simulink model "rgb_conterller_demo"  (Simulink 7.3)
settings: Solver=ode3  SolverMode=SingleTasking  StartTime=0.0  StopTime=10.0  RelTol=1e-3
PreLoadFcn:
  | waijung.modelPreload; % Required for working with Waijung Blockset. Do not remove.
undefined symbols (not defined in the file): CONFIG_GPIO_AS_PINRESET, CONFIG_NFCT_PINS_AS_GPIOS, FLOAT_ABI_HARD, In1, In2, NRF52, NRF52832_XXAA, nRF52832QFAA, NRF52_PAN_74, Out1, Out2, S132, SOFTDEVICE_PRESENT, SWI_DISABLE0, v6
libraries: simulink x1, nrf5_rgb_conterller_lib x1, nrf5_device_config_lib x1
CloseFcn:
  | waijung.modelClose; % Required for working with Waijung Blockset. Do not remove.
settings Model: Creator=Navy  LastModifiedBy=Navy
settings OptimizationCC: OptimizeModelRefInitCode=on  LifeSpan=1
settings HardwareCC: ProdEndianess=LittleEndian  ProdHWDeviceType=ARM Compatible->Cortex - M0  TargetEndianess=LittleEndian  TargetHWDeviceType=ARM Compatible->Cortex - M0
settings RTWCC: SystemTargetFile=nrf5.tlc  GenerateMakefile=off  TemplateMakefile=ert_default_tmf  Description=nRF5 Target  ProcessScript=nrf5_make_rtw_hook
settings CodeAppCC: IgnoreCustomStorageClasses=off
settings STFCustomTargetCC: ModelReferenceCompliant=off  CombineOutputUpdateFcns=on  ERTCustomFileBanners=on  SupportContinuousTime=off  SupportNonInlinedSFcns=off  SystemTargetFile=nrf5.tlc
settings ERTTargetCC: MultiwordLength=2048  ModelReferenceCompliant=off  ParMdlRefBuildCompliant=off  CompOptLevelCompliant=off  ERTFirstTimeCompliant=off  ModelStepFunctionPrototypeControlCompliant=off  CPPClassGenCompliant=off  InlinedParameterPlacement=NonHierarchical  ERTSrcFileBannerTemplate=nrf5_code_template.cgt  ERTHdrFileBannerTemplate=nrf5_code_template.cgt  ERTDataSrcFileTemplate=nrf5_code_template.cgt  ERTDataHdrFileTemplate=nrf5_code_template.cgt  ERTCustomFileTemplate=nrf5_file_process.tlc

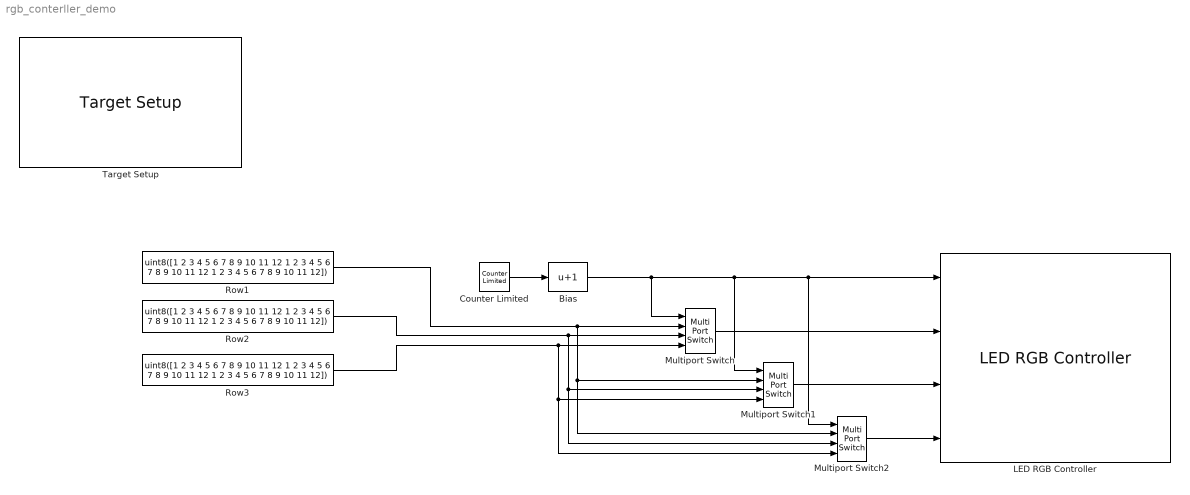
== system rgb_conterller_demo ==
  Bias : Bias  Bias=1
  Counter Limited : simulink/Sources/Counter Limited  SystemSampleTime=-1  uplimit=2  tsamp=-1
  LED RGB Controller : nrf5_rgb_conterller_lib/LED RGB Controller  conf=output  clock=500kHz  panelcount=3  redpin=11  greenpin=12  bluepin=7  clockpin=8  latchpin=5  rowselecta=10  rowselectb=9  portpinstr=0  enablecustomportlabel=off  cinputportlabel=In1,In2  coutputportlabel=Out1,Out2  sampletime=-1  blockid=LEDRGBController  inputporttype=[3 3 3 3]  inputportwidth=[1 36 36 36]  inputportlabel={'Row','R','G','B'}  outputporttype=[]  outputportwidth=[]  outputportlabel={}  compat=0  optionstring="[\"8\",\"11\",\"12\",\"7\",\"5\",\"10\",\"9\",\"3\"]"
  Multiport Switch : MultiPortSwitch  OutDataType=fixdt(1, 16)  OutScaling=2^0
  Multiport Switch1 : MultiPortSwitch  OutDataType=fixdt(1, 16)  OutScaling=2^0
  Multiport Switch2 : MultiPortSwitch  OutDataType=fixdt(1, 16)  OutScaling=2^0
  Row1 : Constant  Value=uint8([1 2 3 4 5 6 7 8 9 10 11 12 1 2 3 4 5 6 7 8 9 10 11 12 1 2 3 4 5 6 7 8 9 10 11 12])  OutDataType=fixdt(1, 16)  OutScaling=2^0
  Row2 : Constant  Value=uint8([1 2 3 4 5 6 7 8 9 10 11 12 1 2 3 4 5 6 7 8 9 10 11 12 1 2 3 4 5 6 7 8 9 10 11 12])  OutDataType=fixdt(1, 16)  OutScaling=2^0
  Row3 : Constant  Value=uint8([1 2 3 4 5 6 7 8 9 10 11 12 1 2 3 4 5 6 7 8 9 10 11 12 1 2 3 4 5 6 7 8 9 10 11 12])  OutDataType=fixdt(1, 16)  OutScaling=2^0
  Target Setup : nrf5_device_config_lib/Target Setup  Priority=100  compiler=GNU ARM  previous_compiler=GNU ARM  mcu=nRF52832QFAA (S132-v6)  family=nrf52  softdevice=S132  clockconfig=None  system_nrf5_c_path=c:\users\Krisada\desktop\waijung\waijung-subversion-trunk\targets\nrf5_target\nrf5\utils\nrf5_lib\inc  lowpower=off  showmemoryconfiguration=on  stacksize=0xC00  heapsize=0x00  enableautocompiledownload=on  fullchiperase=off  ble_secure_dfu=off  ble_secure_dfu_public_key='123bd49bffb387f1de3dc8dc1fc8fcce952739d331fafeb7dd16837154ace7994a0a05af319f68e2a07478477b8db746643d6dd7f5f191193738984ffcd2b963'  programmerinterface=aMG USB Connect  editctrlstr=on  compilercontrolstr=-O3 -g3 -mcpu=cortex-m4 -mthumb -mabi=aapcs -Wall -mfloat-abi=hard -mfpu=fpv4-sp-d16 -ffunction-sections -fdata-sections -fno-strict-aliasing -fno-builtin -fshort-enums  assemblercontrolstr=-O3 -g3 -mcpu=cortex-m4 -mthumb -mabi=aapcs -mfloat-abi=hard -mfpu=fpv4-sp-d16  linkercontrolstr=-O3 -g3 -mthumb -mabi=aapcs -mcpu=cortex-m4 -mfloat-abi=hard -mfpu=fpv4-sp-d16 -Wl,--gc-sections --specs=nano.specs  global_define=CONFIG_GPIO_AS_PINRESET,FLOAT_ABI_HARD,NRF52,NRF52832_XXAA,NRF52_PAN_74,S132,SOFTDEVICE_PRESENT,SWI_DISABLE0,CONFIG_NFCT_PINS_AS_GPIOS  runafterdownload=on  execprofile=None  profileruart=3  profilerbaud=500000  profilertxpin=D8  profilerinitstr=0.01,168000000,1680000,500000,0  manualsetsampletime=on  sampletime=0.1  blockid=TargetSetup  systickreloadvalue=10  hseval=8000000  lastprofileruart=3  hclk=168000000  flashorigin=0x26000  flashlength=256k  ramorigin=0x200032C8  ramlength=51k  useextram=off  optionstring="[\"s132\",\"off\"]"
  wires:
  Multiport Switch/1 -> LED RGB Controller/2
  Multiport Switch1/1 -> LED RGB Controller/3
  Multiport Switch2/1 -> LED RGB Controller/4
  Counter Limited/1 -> Bias/1
  Row1/1 -> Multiport Switch/2, Multiport Switch1/2, Multiport Switch2/2
  Row2/1 -> Multiport Switch/3, Multiport Switch1/3, Multiport Switch2/3
  Row3/1 -> Multiport Switch/4, Multiport Switch1/4, Multiport Switch2/4
  Bias/1 -> Multiport Switch1/1, Multiport Switch2/1, LED RGB Controller/1, Multiport Switch/1
